simulink model "AE432_FinDel_Pioneer_WayPoint_Sim_2018a"  (R2018a)
settings: Solver=VariableStepAuto  StartTime=0  StopTime=445  FixedStep=T  RelTol=1e-3  EnableMultiTasking=on
InitFcn:
  | Waypoints
  | RollPitchTracking_Stab_ControlPioneer
values from neighbouring files (symbols this model uses):
  h = 220*ones(1,36)    [Waypoints.m]
  K1 = place(Along,Blong,P1)    [RollPitchTracking_Stab_ControlPioneer.m]
  T = 0.05    [Waypoints.m]
  x = [0 250 250 250 250 250 1250 2250 2150 2100 2050 2000 1900 1250 1250 500 500 500 500 1500 2250 2250 2250 2250 1000 1000 1000 1000 1250 1250 1250 1250 1750 1750 1750 1750]    [Waypoints.m]
  y = [0 1250 1750 2750 3500 4250 4250 4250 3750 3000 1750 1250 250 250 1500 2500 3000 3500 4000 4000 4000 3500 3000 2500 2500 3000 3500 4000 4000 3500 3000 2500 2500 3000 3500 4000]    [Waypoints.m]
undefined symbols (not defined in the file or in its folder): DiscIntNeverNeededParam, Td
libraries: simulink x19, simulink_extras x10, aerolibfltsims x2, airlib x1, aerolibanimutils x1
(part 1 of 2)
settings Model: Creator=VERBERNJ  LastModifiedBy=SHETTYA1
settings DataIOCC: SaveFormat=Array  SignalLoggingSaveFormat=ModelDataLogs  SaveOutput=off  SaveTime=off
settings OptimizationCC: BlockReduction=off  BooleanDataType=off  InitFltsAndDblsToZero=on
settings DebuggingCC: SaveWithParameterizedLinksMsg=none  UnderspecifiedInitializationDetection=Classic  MergeDetectMultiDrivingBlocksExec=none  SignalResolutionControl=TryResolveAllWithWarning  MultiTaskDSMMsg=warning  MultiTaskCondExecSysMsg=none  LibraryContextMissingDiagnostic=warning
settings HardwareCC: TargetUnknown=on
settings ModelReferenceCC: PropagateSignalLabelsOutOfModel=off
settings SFSimCC: SimUseLocalCustomCode=on
settings RTWCC: RTWUseLocalCustomCode=on
settings GRTTargetCC: TargetFcnLib=ansi_tfl_tmw.mat  TargetLangStandard=C89/C90 (ANSI)  CombineOutputUpdateFcns=off  GRTInterface=on

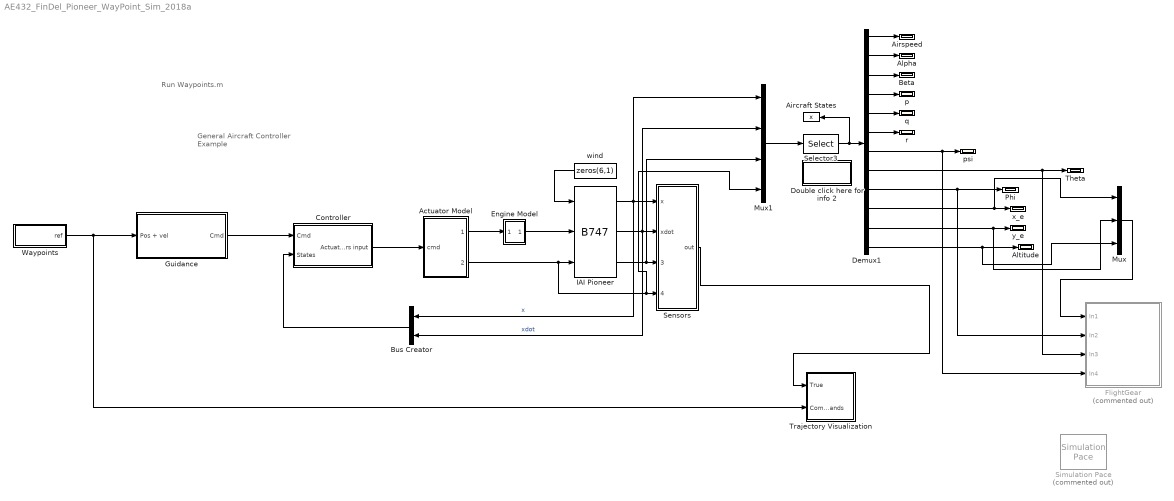
== system AE432_FinDel_Pioneer_WayPoint_Sim_2018a ==
  note: Run Waypoints.m
  note: General Aircraft
      | Controller Example
  " IAI Pioneer " : airlib/B747  GM1="[0.5486  5.1511  2.8261   47.2259  90.9483  111.4754   0  -6.6462  0   190.512]"  CD_wind="[0.060  0.430  0  0.0180  0]"  CL_wind="[0.385  4.78  8.05  0.401  0]"  Cm_body="[0.194  -2.12   -36.6   -1.76    0]"  CY_body="[0   -0.819    0     0    0.191    0]"  Cl_body="[0   -0.023   -0.450   0.265   -0.161  -0.00229]"  Cn_body="[0    0.109  -0.110  -0.200    0.0200  -0.0917]"  x0="[41.1556 0.0506 0   0 0 0   0 0.0506 0   0 0 220]"
  Actuator Model : Subsystem
  Aircraft States : ToWorkspace  VariableName=x  SampleTime=0.05
  Airspeed : Scope
  Alpha : Scope
  Altitude : Scope
  Beta : Scope
  Bus Creator : BusCreator  Inputs=2
  Controller : Subsystem
  Demux1 : Demux  Outputs=12
  Double click here for info 2 : Subsystem
      mask Display: disp('Output\nSignals')
  Engine Model : Subsystem
  FlightGear : Subsystem  Commented=on
  Guidance : Subsystem
  Mux : Mux  Inputs=3
  Mux1 : Mux  Inputs=[12 12 12 4]
  Phi : Scope
  Selector3 : Selector  InputPortWidth=40  IndexOptions=Index vector (dialog)  Indices=1:12  OutputSizes=1
  Sensors : Subsystem
  Simulation Pace : aerolibanimutils/Simulation Pace  Commented=on  SimulationPace=1  SleepMode=MATLAB Thread  OutputPaceError=off  SampleTime=Td
      settings: AttributesFormatString=%<SimulationPace> sec/sec
  Theta : Scope
  Trajectory Visualization : Subsystem
  Waypoints : Subsystem  mask(Reference Path Generation){Px=y, Py=x, Ph=h, Pt=t, T=T}
      mask prompts: Px "X Positions"; Py "Y Positions"; Ph "H Positions"; Pt "Time"; T "Sample Time"
      mask help:
      | This block generates a 3D trajectory. The output is a vector containing
      |   the position and velocity of a point that sequentially visits each X,Y,Z
      |   position at the corrisponding time. The velocity is constant between
      |   one visited point and the next.
      mask Help:
      | This block generates a 3D trajectory. The output is a vector containing
      |   the position and velocity of a point that sequentially visits each X,Y,Z
      |   position at the corrisponding time. The velocity is constant between
      |   one visited point and the next.
  p : Scope
  psi : Scope
  q : Scope
  r : Scope
  wind : Constant  Value=zeros(6,1)
  x_e : Scope
  y_e : Scope
  wires:
  " IAI Pioneer "/1 -> Mux1/1, Bus Creator/1, Sensors/1(x)  "x"
  wind/1 -> " IAI Pioneer "/1
  Actuator Model/1(Throttle) -> Engine Model/1(uprop)
  " IAI Pioneer "/2 -> Mux1/2, Bus Creator/2, Sensors/2(xdot)  "xdot"
  " IAI Pioneer "/3 -> Mux1/3, Sensors/3(others)
  Actuator Model/2(Surfaces) -> " IAI Pioneer "/3, Mux1/4, Sensors/4(controls)
  Waypoints/1(ref) -> Guidance/1(Pos + vel), Trajectory Visualization/2(Commands)
  Sensors/1(out) -> Trajectory Visualization/1(True)
  Engine Model/1(FMprop) -> " IAI Pioneer "/2
  Controller/1(Actuators input) -> Actuator Model/1(cmd)
  Guidance/1(Cmd) -> Controller/1(Cmd)
  Bus Creator/1 -> Controller/2(States)
  Demux1/12 -> Mux/3, Altitude/1
  Demux1/11 -> Mux/2, y_e/1
  Demux1/10 -> Mux/1, x_e/1
  Demux1/8 -> FlightGear/3(In3), Theta/1
  Demux1/7 -> FlightGear/4(In4), psi/1
  Demux1/6 -> r/1
  Demux1/5 -> q/1
  Demux1/4 -> p/1
  Demux1/3 -> Beta/1
  Demux1/2 -> Alpha/1
  Demux1/1 -> Airspeed/1
  Selector3/1 -> Aircraft States/1, Demux1/1
  Mux1/1 -> Selector3/1
  Demux1/9 -> Phi/1, FlightGear/2(In2)
  Mux/1 -> FlightGear/1(In1)

== system AE432_FinDel_Pioneer_WayPoint_Sim_2018a/Actuator Model ==
  cmd : Inport
  Demux : Demux  Outputs=[1 1 1 1]
  Elevator Trim : Constant  Value=0.0493
  Mux1 : Mux
  Sum5 : Sum  Inputs=++|  SaturateOnIntegerOverflow=on  InputSameDT=on  OutDataTypeStr=Inherit: Same as first input
  Thrust : Constant  Value=0.36
  flap : Constant  Value=0
  wind1 : Gain  Gain=-1  SaturateOnIntegerOverflow=on  OutDataTypeStr=Inherit: Same as input  ParamDataTypeStr=Inherit: Same as input
  wind2 : Gain  Gain=-1/3  SaturateOnIntegerOverflow=on  OutDataTypeStr=Inherit: Same as input  ParamDataTypeStr=Inherit: Same as input
  wind4 : Gain  Gain=-1/3  SaturateOnIntegerOverflow=on  OutDataTypeStr=Inherit: Same as input  ParamDataTypeStr=Inherit: Same as input
  Throttle : Outport
  Surfaces : Outport  Port=2
  wires:
  flap/1 -> Mux1/4
  cmd/1 -> Demux/1
  Mux1/1 -> Surfaces/1  "uaero"
  Demux/2 -> wind2/1
  Demux/3 -> wind4/1
  Demux/1 -> wind1/1
  Elevator Trim/1 -> Sum5/1
  Sum5/1 -> Mux1/1
  wind2/1 -> Mux1/2
  wind4/1 -> Mux1/3
  wind1/1 -> Sum5/2
  Demux/4 -> Throttle/1

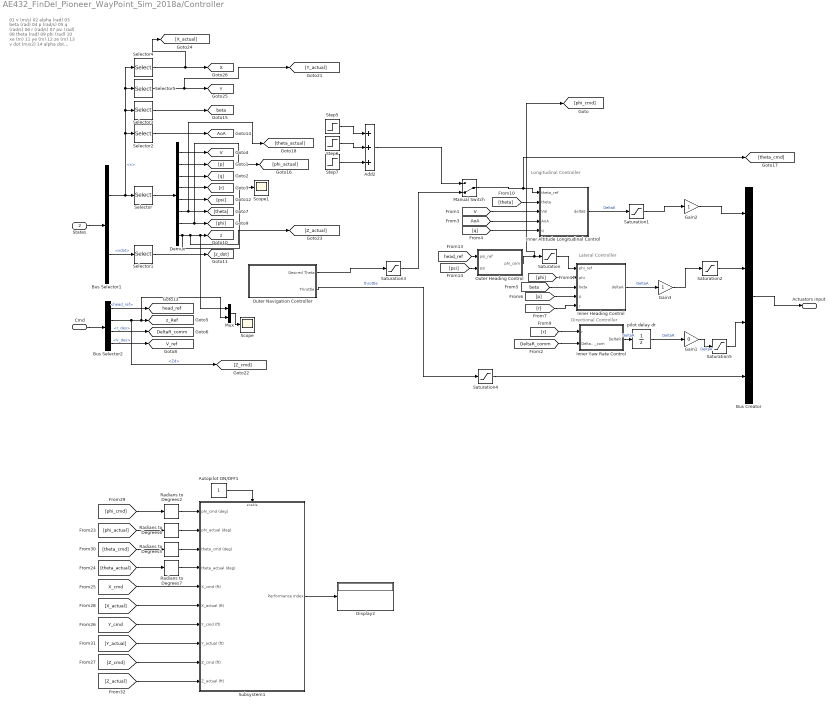
== system AE432_FinDel_Pioneer_WayPoint_Sim_2018a/Controller ==
  note: 01 v (m/s)
      | 02 alpha (rad)
      | 03 beta (rad)
      | 04 p (rad/s)
      | 05 q (rad/s)
      | 06 r  (rad/s)
      | 07 psi (rad)
      | 08 theta (rad)
      | 09 phi (rad)
      | 10 xe (m)
      | 11 ye (m)
      | 12 ze (m)
      |
      | 13 v dot (m/s2)
      | 14 alpha dot (rad/s)
      | 15 beta dot (rad/s)
      | 16 p dot (rad/s2)
      | 17 q dot (rad/s2)
      | 18 r dot (rad/s2)
      | 19 fi dot (rad/s)
      | 20 theta dot (rad/s)
      | 21 psi dot (rad/s)
      | 22 xe dot (m/s)
      | 23 ye dot (m/s)
      | 24 ze dot (m/s)
      |
      | 25 u dot (m/s2)
      | 26 v dot (m/s2)
      | 27 w dot (m/s2)
      | 28 pb/2v (rad)
      | 29 qc/v (rad)
      | 30 rb/v (rad)
      | 31 Ax (g)
      | 32 Ay (g)
      | 33 Az (g)
      | 34 ax (g)
      | 35 ay (g)
      | 36 az (g)
  note: Directional Controller
  note: Longitudinal Controller
  note: Lateral Controller
  Cmd : Inport
  States : Inport  Port=2
  Add2 : Sum  Inputs=+++
  Autopilot ON/OFF1 : Constant
  Bus Creator : BusCreator  Inputs=4
  Bus Selector1 : BusSelector  OutputSignals=x,xdot
  Bus Selector2 : BusSelector  OutputSignals=head_ref,Zd,r_des,V_des
  Demux : Demux  Outputs=8
  Display2 : Display
  Gain1 : Gain  Gain=0
  Gain2 : Gain
  Gain3 : Gain
  Inner Altitude Longitudinal Control : Subsystem  TreatAsAtomicUnit=on
  Inner Heading Control : Subsystem  TreatAsAtomicUnit=on
  Inner Yaw Rate Control : Subsystem  TreatAsAtomicUnit=on
  Manual Switch : ManualSwitch  CurrentSetting=0
  Mux : Mux  Inputs=2
  Outer Heading Control : Subsystem  TreatAsAtomicUnit=on
  Outer Navigation Controller : Subsystem
  Radians to Degrees{2,5..7} (4 alike) : simulink_extras/Transformations/Radians to Degrees
  Saturation : Saturate  UpperLimit=62*pi/180  LowerLimit=-62*pi/180
  Saturation1 : Saturate  UpperLimit=40*pi/180  LowerLimit=-40*pi/180
  Saturation2 : Saturate  UpperLimit=45*pi/180  LowerLimit=-45*pi/180
  Saturation3 : Saturate  UpperLimit=65*pi/180  LowerLimit=-65*pi/180
  Saturation4 : Saturate  UpperLimit=1  LowerLimit=0
  Saturation5 : Saturate  UpperLimit=40*pi/180  LowerLimit=-40*pi/180
  Scope : Scope
  Scope1 : Scope
  Selector : Selector  InputPortWidth=12  IndexOptions=Index vector (dialog)  Indices=[1 4 5 6 7 8 9 12]  OutputSizes=1
  Selector1 : Selector  InputPortWidth=12  IndexOptions=Index vector (dialog)  Indices=12  OutputSizes=1
  Selector2 : Selector  InputPortWidth=12  IndexOptions=Index vector (dialog)  Indices=2  OutputSizes=1
  Selector3 : Selector  InputPortWidth=12  IndexOptions=Index vector (dialog)  Indices=3  OutputSizes=1
  Selector4 : Selector  InputPortWidth=12  IndexOptions=Index vector (dialog)  Indices=10  OutputSizes=1
  Selector5 : Selector  InputPortWidth=12  IndexOptions=Index vector (dialog)  Indices=11  OutputSizes=1
  Step5 : Step  After=30*pi/180
  Step6 : Step  Time=20  Before=30*pi/180  After=-30*pi/180
  Step7 : Step  Time=40  Before=-30*pi/180  After=0
  Subsystem1 : Subsystem
  pilot delay dr : UnitDelay  SampleTime=-1
  Actuators input : Outport
  tag scope: AoA=global, DeltaR_comm=global, V=global, V_ref=global, X=global, Y=global, beta=global, head_ref=global, z=global, z_Ref=global
  wires:
  Bus Selector1/2 -> Selector1/1  "<xdot>"
  Selector/1 -> Demux/1
  Bus Selector1/1 -> Selector5/1, Selector4/1, Selector3/1, Selector2/1, Selector/1  "<x>"
  Outer Navigation Controller/2(Throttle) -> Saturation4/1  "throttle"
  pilot delay dr/1 -> Gain1/1  "DeltaR"
  Demux/1 -> [V]
  Inner Yaw Rate Control/1(DeltaR) -> pilot delay dr/1  "DeltaR"
  [DeltaR_comm] -> Inner Yaw Rate Control/2(DeltaR_com)
  [theta] -> Inner Altitude Longitudinal Control/2(theta)
  [phi] -> Inner Heading Control/2(phi)
  [psi] -> Outer Heading Control/2(psi)
  [head_ref] -> Outer Heading Control/1(psi_ref)
  Bus Selector2/4 -> [V_ref]  "<V_des>"
  Bus Selector2/3 -> [DeltaR_comm]  "<r_des>"
  Bus Selector2/2 -> [Z_cmd], Mux/2, [z_Ref]  "<Zd>"
  Bus Selector2/1 -> [head_ref]  "<head_ref>"
  Demux/5 -> [psi]
  [r] -> Inner Yaw Rate Control/1(r)
  States/1 -> Bus Selector1/1
  Selector1/1 -> [z_dot]
  Demux/8 -> Scope1/1, [Z_actual], Mux/1, [z]
  Demux/7 -> [phi_actual], [phi]
  Demux/4 -> [r]
  Demux/3 -> [q]
  Demux/2 -> [p]
  Bus Creator/1 -> Actuators input/1
  Cmd/1 -> Bus Selector2/1
  Manual Switch/1 -> [theta_cmd], Inner Altitude Longitudinal Control/1(theta_ref)
  [V] -> Inner Altitude Longitudinal Control/3(Vel)
  [AoA] -> Inner Altitude Longitudinal Control/4(AoA)
  [q] -> Inner Altitude Longitudinal Control/5(q)
  Selector2/1 -> [AoA]
  Selector3/1 -> [beta]
  Gain1/1 -> Saturation5/1  "DeltaR"
  Inner Heading Control/1(deltaA) -> Gain3/1  "DeltaA"
  Gain2/1 -> Bus Creator/1
  [beta] -> Inner Heading Control/3(beta)
  [p] -> Inner Heading Control/4(p)
  [r] -> Inner Heading Control/5(r)
  Add2/1 -> Manual Switch/1
  Step6/1 -> Add2/2
  Step5/1 -> Add2/1
  Step7/1 -> Add2/3
  Outer Heading Control/1(phi_com) -> Saturation/1, [phi_cmd]
  Saturation/1 -> Inner Heading Control/1(phi_ref)
  Saturation1/1 -> Gain2/1
  Inner Altitude Longitudinal Control/1(deltaE) -> Saturation1/1  "DeltaE"
  Saturation2/1 -> Bus Creator/2
  Gain3/1 -> Saturation2/1
  Saturation3/1 -> Manual Switch/2
  Outer Navigation Controller/1(Desired Theta) -> Saturation3/1
  Demux/6 -> [theta_actual], [theta]
  Selector5/1 -> [Y_actual], [Y]
  Selector4/1 -> [X_actual], [X]
  Mux/1 -> Scope/1
  Saturation4/1 -> Bus Creator/4
  Saturation5/1 -> Bus Creator/3
  Radians to Degrees5/1 -> Subsystem1/3(theta_cmd (deg))
  [X_actual] -> Subsystem1/6(X_actual (ft))
  Radians to Degrees7/1 -> Subsystem1/4(theta_actual (deg))
  [Y_actual] -> Subsystem1/8(Y_actual (ft))
  [Z_actual] -> Subsystem1/10(Z_actual (ft))
  [phi_cmd] -> Radians to Degrees2/1
  [phi_actual] -> Radians to Degrees6/1
  [theta_cmd] -> Radians to Degrees5/1
  [Y_cmd] -> Subsystem1/7(Y_cmd (ft))
  Radians to Degrees6/1 -> Subsystem1/2(phi_actual (deg))
  [X_cmd] -> Subsystem1/5(X_cmd (ft))
  Radians to Degrees2/1 -> Subsystem1/1(phi_cmd (deg))
  Autopilot ON/OFF1/1 -> Subsystem1/Enable
  Subsystem1/1(Performance Index) -> Display2/1
  [Z_cmd] -> Subsystem1/9(Z_cmd (ft))
  [theta_actual] -> Radians to Degrees7/1

== system AE432_FinDel_Pioneer_WayPoint_Sim_2018a/Double click here for info 2 ==
  note: 01 v (m/s)
      | 02 alpha (rad)
      | 03 beta (rad)
      | 04 p (rad/s)
      | 05 q (rad/s)
      | 06 r  (rad/s)
      | 07 psi (rad)
      | 08 theta (rad)
      | 09 phi (rad)
      | 10 xe (m)
      | 11 ye (m)
      | 12 ze (m)
      | 13 v dot (m/s2)
      | 14 alpha dot (rad/s)
      | 15 beta dot (rad/s)
      | 16 p dot (rad/s2)
      | 17 q dot (rad/s2)
      | 18 r dot (rad/s2)
      | 19 fi dot (rad/s)
      | 20 theta dot (rad/s)
      | 21 psi dot (rad/s)
      | 22 xe dot (m/s)
      | 23 ye dot (m/s)
      | 24 ze dot (m/s)
      | 25 u dot (m/s2)
      | 26 v dot (m/s2)
      | 27 w dot (m/s2)
      | 28 pb/2v (rad)
      | 29 qc/v (rad)
      | 30 rb/v (rad)
      | 31 Ax (g)
      | 32 Ay (g)
      | 33 Az (g)
      | 34 ax (g)
      | 35 ay (g)
      | 36 az (g)
      | 37 delta elevators (rad)
      | 38 delta ailerons (rad)
      | 39 delta rudder (rad)
      | 40 delta stabs (rad)

== system AE432_FinDel_Pioneer_WayPoint_Sim_2018a/Engine Model ==
  uprop : Inport
  Mux1 : Mux  Inputs=6
  const : Constant  Value=0  SampleTime=-1
  xfix : Gain  Gain=667  SaturateOnIntegerOverflow=on  OutDataTypeStr=Inherit: Same as input  ParamDataTypeStr=Inherit: Same as input
  FMprop : Outport  InitialOutput=0
  wires:
  uprop/1 -> xfix/1
  Mux1/1 -> FMprop/1
  const/1 -> Mux1/5, Mux1/4, Mux1/3, Mux1/2, Mux1/6
  xfix/1 -> Mux1/1

== system AE432_FinDel_Pioneer_WayPoint_Sim_2018a/FlightGear ==
  In1 : Inport
  In2 : Inport  Port=2
  In3 : Inport  Port=3
  In4 : Inport  Port=4
  Data Type Conversion : DataTypeConversion  OutDataTypeStr=single
  Data Type Conversion1 : DataTypeConversion  OutDataTypeStr=single
  Data Type Conversion2 : DataTypeConversion  OutDataTypeStr=single
  Lat,Lon,Elev Convertor : Subsystem
  Pack net_fdm Packet for FlightGear : aerolibfltsims/Pack net_fdm Packet for FlightGear  FlightGearVersion=v2.4  ShowPositionAttitudeInputs=on  ShowVelocityAccelerationInputs=off  ShowControlSurfacePositionInputs=off  ShowEngineFuelInputs=off  ShowLandingGearInputs=off  ShowEnvironmentInputs=off  SampleTime=-1
      settings: SourceProductName=Aerospace Blockset  SourceProductBaseCode=AE
  Send net_fdm Packet to FlightGear : aerolibfltsims/Send net_fdm Packet to FlightGear  DestinationIpAddress=127.0.0.1  DestinationPort=5502  LocalIpPort=-1  varLen=off  SampleTime=-1
      settings: SourceProductName=Aerospace Blockset  SourceProductBaseCode=AE
  wires:
  In2/1 -> Data Type Conversion2/1
  In3/1 -> Data Type Conversion1/1
  Lat,Lon,Elev Convertor/2(Lat) -> Pack net_fdm Packet for FlightGear/2
  Lat,Lon,Elev Convertor/3(Ele) -> Pack net_fdm Packet for FlightGear/3
  In1/1 -> Lat,Lon,Elev Convertor/1(Inp)
  Data Type Conversion1/1 -> Pack net_fdm Packet for FlightGear/5
  Data Type Conversion2/1 -> Pack net_fdm Packet for FlightGear/4
  Lat,Lon,Elev Convertor/1(Lon) -> Pack net_fdm Packet for FlightGear/1
  In4/1 -> Data Type Conversion/1
  Data Type Conversion/1 -> Pack net_fdm Packet for FlightGear/6
  Pack net_fdm Packet for FlightGear/1 -> Send net_fdm Packet to FlightGear/1

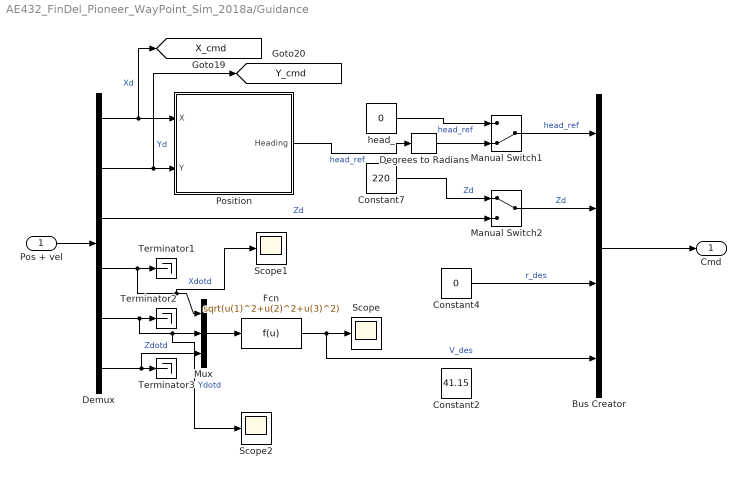
== system AE432_FinDel_Pioneer_WayPoint_Sim_2018a/Guidance ==
  Pos + vel : Inport
  Bus Creator : BusCreator  Inputs=4
  Constant2 : Constant  Value=41.15  SampleTime=-1
  Constant4 : Constant  Value=0  SampleTime=-1
  Constant7 : Constant  Value=220  SampleTime=-1
  Degrees to Radians : simulink_extras/Transformations/Degrees to Radians
  Demux : Demux  Outputs=6
  Fcn : Fcn  Expr=sqrt(u(1)^2+u(2)^2+u(3)^2)
  Manual Switch1 : ManualSwitch  CurrentSetting=0
  Manual Switch2 : ManualSwitch
  Mux : Mux  Inputs=3
  Position : Subsystem
  Scope : Scope
  Scope1 : Scope
  Scope2 : Scope
  Terminator1 : Terminator
  Terminator2 : Terminator
  Terminator3 : Terminator
  head_ : Constant  Value=0  SampleTime=-1
  Cmd : Outport
  tag scope: X_cmd=global, Y_cmd=global
  wires:
  Pos + vel/1 -> Demux/1
  Demux/3 -> Manual Switch2/2  "Zd"
  Bus Creator/1 -> Cmd/1
  Degrees to Radians/1 -> Manual Switch1/2
  head_/1 -> Manual Switch1/1  "head_ref"
  Position/1(Heading) -> Degrees to Radians/1  "head_ref"
  Demux/4 -> Scope1/1, Mux/1, Terminator1/1  "Xdotd"
  Manual Switch2/1 -> Bus Creator/2  "Zd"
  Manual Switch1/1 -> Bus Creator/1  "head_ref"
  Demux/6 -> Mux/3, Terminator3/1  "Zdotd"
  Fcn/1 -> Bus Creator/4, Scope/1  "V_des"
  Constant4/1 -> Bus Creator/3  "r_des"
  Demux/2 -> [Y_cmd], Position/2(Y)  "Yd"
  Constant7/1 -> Manual Switch2/1  "Zd"
  Demux/1 -> [X_cmd], Position/1(X)  "Xd"
  Demux/5 -> Scope2/1, Mux/2, Terminator2/1  "Ydotd"
  Mux/1 -> Fcn/1

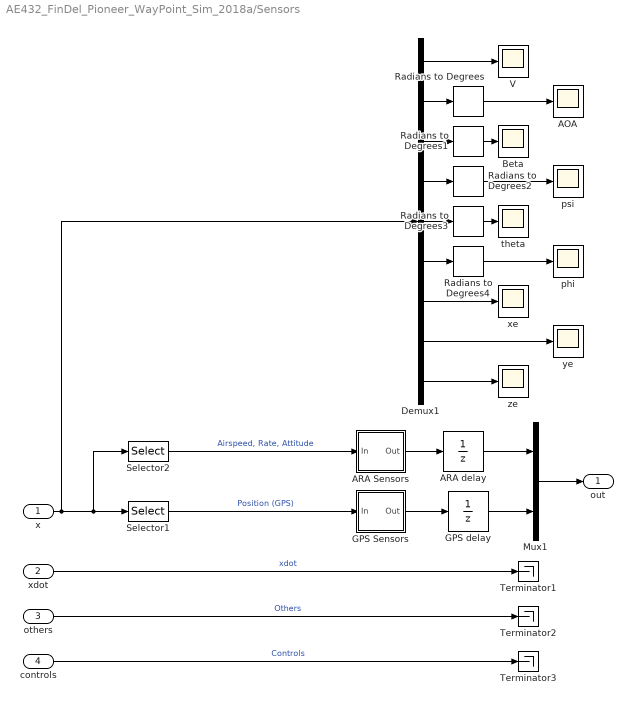
== system AE432_FinDel_Pioneer_WayPoint_Sim_2018a/Sensors ==
  x : Inport
  xdot : Inport  Port=2
  others : Inport  Port=3
  controls : Inport  Port=4
  AOA : Scope
  ARA Sensors : Subsystem
  ARA delay : UnitDelay  InitialCondition="[60 -0.0293682 0   0 0 0   0 -0.0293682 0]"  SampleTime=T
  Beta : Scope
  Demux1 : Demux  Outputs=9
  GPS Sensors : Subsystem
  GPS delay : UnitDelay  InitialCondition="[-2.5  0  60]"  SampleTime=T
  Mux1 : Mux  Inputs=[9 3]
  Radians to Degrees{,1..4} (5 alike) : simulink_extras/Transformations/Radians to Degrees
  Selector1 : Selector  InputPortWidth=12  IndexOptions=Index vector (dialog)  Indices=[10 11 12]  OutputSizes=1
  Selector2 : Selector  InputPortWidth=12  IndexOptions=Index vector (dialog)  Indices=[1:9]  OutputSizes=1
  Terminator1 : Terminator
  Terminator2 : Terminator
  Terminator3 : Terminator
  V : Scope
  phi : Scope
  psi : Scope
  theta : Scope
  xe : Scope
  ye : Scope
  ze : Scope
  out : Outport
  wires:
  controls/1 -> Terminator3/1  "Controls"
  others/1 -> Terminator2/1  "Others"
  xdot/1 -> Terminator1/1  "xdot"
  Mux1/1 -> out/1
  GPS Sensors/1(Out) -> GPS delay/1
  GPS delay/1 -> Mux1/2
  ARA delay/1 -> Mux1/1
  Selector1/1 -> GPS Sensors/1(In)  "Position (GPS)"
  ARA Sensors/1(Out) -> ARA delay/1
  Selector2/1 -> ARA Sensors/1(In)  "Airspeed, Rate, Attitude"
  x/1 -> Demux1/1, Selector2/1, Selector1/1
  Radians to Degrees1/1 -> Beta/1
  Radians to Degrees4/1 -> phi/1
  Demux1/8 -> ye/1
  Radians to Degrees2/1 -> psi/1
  Demux1/4 -> Radians to Degrees2/1
  Demux1/2 -> Radians to Degrees/1
  Demux1/9 -> ze/1
  Demux1/3 -> Radians to Degrees1/1
  Radians to Degrees/1 -> AOA/1
  Demux1/6 -> Radians to Degrees4/1
  Demux1/5 -> Radians to Degrees3/1
  Demux1/1 -> V/1
  Radians to Degrees3/1 -> theta/1
  Demux1/7 -> xe/1

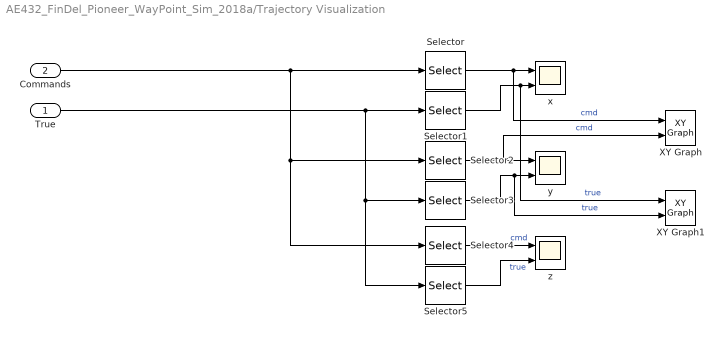
== system AE432_FinDel_Pioneer_WayPoint_Sim_2018a/Trajectory Visualization ==
  True : Inport
  Commands : Inport  Port=2
  Selector : Selector  InputPortWidth=6  IndexOptions=Index vector (dialog)  Indices=1  OutputSizes=1
  Selector1 : Selector  InputPortWidth=12  IndexOptions=Index vector (dialog)  Indices=10  OutputSizes=1
  Selector2 : Selector  InputPortWidth=6  IndexOptions=Index vector (dialog)  Indices=2  OutputSizes=1
  Selector3 : Selector  InputPortWidth=12  IndexOptions=Index vector (dialog)  Indices=11  OutputSizes=1
  Selector4 : Selector  InputPortWidth=6  IndexOptions=Index vector (dialog)  Indices=3  OutputSizes=1
  Selector5 : Selector  InputPortWidth=12  IndexOptions=Index vector (dialog)  Indices=12  OutputSizes=1
  XY Graph : simulink/Sinks/XY Graph  xmin=-100  xmax=5000  ymin=-100  ymax=3000  st=-1
  XY Graph1 : simulink/Sinks/XY Graph  xmin=-100  xmax=5000  ymin=-100  ymax=3000  st=-1
  x : Scope  NumInputPorts=2
  y : Scope  NumInputPorts=2
  z : Scope  NumInputPorts=2
  wires:
  Commands/1 -> Selector/1, Selector4/1, Selector2/1
  Selector1/1 -> XY Graph1/1, x/2  "true"
  Selector/1 -> XY Graph/1, x/1  "cmd"
  Selector2/1 -> XY Graph/2, y/1  "cmd"
  Selector3/1 -> XY Graph1/2, y/2  "true"
  Selector4/1 -> z/1  "cmd"
  Selector5/1 -> z/2  "true"
  True/1 -> Selector1/1, Selector5/1, Selector3/1

== system AE432_FinDel_Pioneer_WayPoint_Sim_2018a/Waypoints ==
  Clock : Clock
  Delay : UnitDelay  InitialCondition=[Px(1) Py(1) Ph(1)]  SampleTime=T
  Derivative : Subsystem  mask(Time Derivative){x0=[Px(1) Py(1) Ph(1)]'-[Px(2)-Px(1) Py(2)-Py(1) Ph(2)-Ph(1)]'/(Pt(2)-Pt(1))*T, T=T}
      mask prompts: x0 "Initial Condition"; T "Sampling Time"
      mask help:
      | First order approximation of the time derivative of the input signal,
      |   the original one is buggy.
  Hd(t) : Lookup  InputValues=Pt  Table=Ph  SaturateOnIntegerOverflow=on
  Horizon Time : Constant  Value=0
  Math Function : Math  Operator=mod  SaturateOnIntegerOverflow=on
  Mux : Mux  Inputs=3
  Mux2 : Mux  Inputs=[3 3]
  Sum2 : Sum  Inputs=++|  SaturateOnIntegerOverflow=on  InputSameDT=on  OutDataTypeStr=Inherit: Same as first input
  Time Limit : Constant  Value=Pt(end)
  Xd(t) : Lookup  InputValues=Pt  Table=Px  SaturateOnIntegerOverflow=on
  Yd(t) : Lookup  InputValues=Pt  Table=Py  SaturateOnIntegerOverflow=on
  ref : Outport
  wires:
  Mux2/1 -> ref/1
  Derivative/1(xdot) -> Mux2/2
  Delay/1 -> Mux2/1
  Xd(t)/1 -> Mux/1
  Yd(t)/1 -> Mux/2
  Hd(t)/1 -> Mux/3
  Sum2/1 -> Math Function/1
  Horizon Time/1 -> Sum2/1
  Clock/1 -> Sum2/2
  Math Function/1 -> Xd(t)/1, Yd(t)/1, Hd(t)/1
  Time Limit/1 -> Math Function/2
  Mux/1 -> Delay/1, Derivative/1(x)

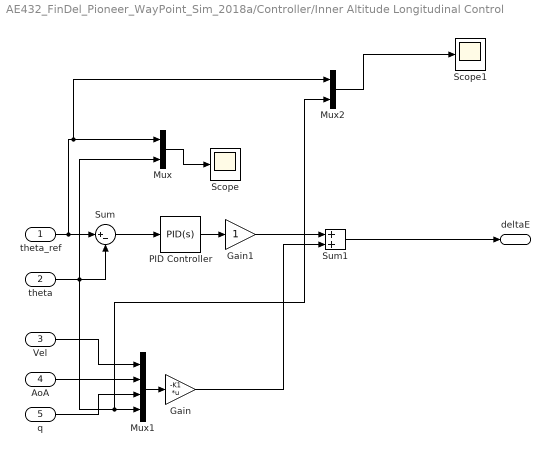
== system AE432_FinDel_Pioneer_WayPoint_Sim_2018a/Controller/Inner Altitude Longitudinal Control ==
  theta_ref : Inport
  theta : Inport  Port=2
  Vel : Inport  Port=3
  AoA : Inport  Port=4
  q : Inport  Port=5
  Gain : Gain  Gain=-K1  Multiplication=Matrix(K*u)
  Gain1 : Gain
  Mux : Mux  Inputs=2
  Mux1 : Mux
  Mux2 : Mux  Inputs=2
  PID Controller : simulink/Continuous/PID Controller  Controller=PID  TimeDomain=Continuous-time  SampleTime=-1  IntegratorMethod=Forward Euler  FilterMethod=Forward Euler  Form=Parallel  UseFilter=on  ControllerParametersSource=internal  P=3.5  I=0.7  D=0.001  N=50  InitialConditionSource=internal  InitialConditionForIntegrator=0  InitialConditionForFilter=0  ExternalReset=none  LimitOutput=off  UpperSaturationLimit=inf  LowerSaturationLimit=-inf  LinearizeAsGain=on  AntiWindupMode=none  Kb=1  TrackingMode=off  Kt=1  PParamMin=[]  PParamMax=[]  IParamMin=[]  IParamMax=[]  DParamMin=[]  DParamMax=[]  NParamMin=[]  NParamMax=[]  KbParamMin=[]  KbParamMax=[]  KtParamMin=[]  KtParamMax=[]  POutMin=[]  POutMax=[]  IOutMin=[]  IOutMax=[]  DOutMin=[]  DOutMax=[]  NOutMin=[]  NOutMax=[]  KbOutMin=[]  KbOutMax=[]  KtOutMin=[]  KtOutMax=[]  IntegratorOutMin=[]  IntegratorOutMax=[]  FilterOutMin=[]  FilterOutMax=[]  SumOutMin=[]  SumOutMax=[]  SumI1OutMin=[]  SumI1OutMax=[]  SumI2OutMin=[]  SumI2OutMax=[]  SumI3OutMin=[]  SumI3OutMax=[]  SumDOutMin=[]  SumDOutMax=[]  SaturationOutMin=[]  SaturationOutMax=[]  IntegratorContinuousStateAttributes=''  IntegratorStateMustResolveToSignalObject=off  IntegratorRTWStateStorageClass=Auto  FilterContinuousStateAttributes=''  FilterStateMustResolveToSignalObject=off  FilterRTWStateStorageClass=Auto  DifferentiatorICPrevScaledInput=0  DifferentiatorOutMin=[]  DifferentiatorOutMax=[]  FilterDiffOutCoefMin=[]  FilterDiffOutCoefMax=[]  SumDenOutMin=[]  SumDenOutMax=[]  SumNumOutMin=[]  SumNumOutMax=[]  ReciprocalOutMin=[]  ReciprocalOutMax=[]  DivideOutMin=[]  DivideOutMax=[]  TunerSelectOption=Transfer Function Based (PID Tuner App)
  Scope : Scope
  Scope1 : Scope
  Sum : Sum  Inputs=|+-
  Sum1 : Sum
  deltaE : Outport
  wires:
  theta/1 -> Mux2/2, Mux1/4, Mux/2, Sum/2
  Sum/1 -> PID Controller/1
  Mux/1 -> Scope/1
  theta_ref/1 -> Mux2/1, Mux/1, Sum/1
  Vel/1 -> Mux1/1
  AoA/1 -> Mux1/2
  q/1 -> Mux1/3
  Mux1/1 -> Gain/1
  PID Controller/1 -> Gain1/1
  Sum1/1 -> deltaE/1
  Gain1/1 -> Sum1/1
  Gain/1 -> Sum1/2
  Mux2/1 -> Scope1/1

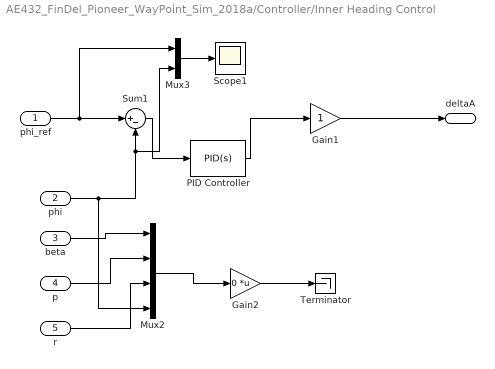
== system AE432_FinDel_Pioneer_WayPoint_Sim_2018a/Controller/Inner Heading Control ==
  phi_ref : Inport
  phi : Inport  Port=2
  beta : Inport  Port=3
  p : Inport  Port=4
  r : Inport  Port=5
  Gain1 : Gain
  Gain2 : Gain  Gain=0  Multiplication=Matrix(K*u)
  Mux2 : Mux
  Mux3 : Mux  Inputs=2
  PID Controller : simulink/Continuous/PID Controller  Controller=PID  TimeDomain=Continuous-time  SampleTime=-1  IntegratorMethod=Forward Euler  FilterMethod=Forward Euler  Form=Parallel  UseFilter=on  ControllerParametersSource=internal  P=2  I=0.355  D=0.025  N=20  InitialConditionSource=internal  InitialConditionForIntegrator=0  InitialConditionForFilter=0  ExternalReset=none  LimitOutput=off  UpperSaturationLimit=inf  LowerSaturationLimit=-inf  LinearizeAsGain=on  AntiWindupMode=none  Kb=1  TrackingMode=off  Kt=1  PParamMin=[]  PParamMax=[]  IParamMin=[]  IParamMax=[]  DParamMin=[]  DParamMax=[]  NParamMin=[]  NParamMax=[]  KbParamMin=[]  KbParamMax=[]  KtParamMin=[]  KtParamMax=[]  POutMin=[]  POutMax=[]  IOutMin=[]  IOutMax=[]  DOutMin=[]  DOutMax=[]  NOutMin=[]  NOutMax=[]  KbOutMin=[]  KbOutMax=[]  KtOutMin=[]  KtOutMax=[]  IntegratorOutMin=[]  IntegratorOutMax=[]  FilterOutMin=[]  FilterOutMax=[]  SumOutMin=[]  SumOutMax=[]  SumI1OutMin=[]  SumI1OutMax=[]  SumI2OutMin=[]  SumI2OutMax=[]  SumI3OutMin=[]  SumI3OutMax=[]  SumDOutMin=[]  SumDOutMax=[]  SaturationOutMin=[]  SaturationOutMax=[]  IntegratorContinuousStateAttributes=''  IntegratorStateMustResolveToSignalObject=off  IntegratorRTWStateStorageClass=Auto  FilterContinuousStateAttributes=''  FilterStateMustResolveToSignalObject=off  FilterRTWStateStorageClass=Auto  DifferentiatorICPrevScaledInput=0  DifferentiatorOutMin=[]  DifferentiatorOutMax=[]  FilterDiffOutCoefMin=[]  FilterDiffOutCoefMax=[]  SumDenOutMin=[]  SumDenOutMax=[]  SumNumOutMin=[]  SumNumOutMax=[]  ReciprocalOutMin=[]  ReciprocalOutMax=[]  DivideOutMin=[]  DivideOutMax=[]  TunerSelectOption=Transfer Function Based (PID Tuner App)
  Scope1 : Scope
  Sum1 : Sum  Inputs=|+-
  Terminator : Terminator
  deltaA : Outport
  wires:
  phi/1 -> Mux2/4, Mux3/2, Sum1/2
  PID Controller/1 -> Gain1/1
  Sum1/1 -> PID Controller/1
  phi_ref/1 -> Mux3/1, Sum1/1
  Mux3/1 -> Scope1/1
  beta/1 -> Mux2/1
  p/1 -> Mux2/2
  r/1 -> Mux2/3
  Mux2/1 -> Gain2/1
  Gain1/1 -> deltaA/1
  Gain2/1 -> Terminator/1

== system AE432_FinDel_Pioneer_WayPoint_Sim_2018a/Controller/Inner Yaw Rate Control ==
  r : Inport
  DeltaR_com : Inport  Port=2
  Gain : Gain
  Mux : Mux  Inputs=2
  PID Controller : simulink/Continuous/PID Controller  Controller=PID  TimeDomain=Continuous-time  SampleTime=-1  IntegratorMethod=Forward Euler  FilterMethod=Forward Euler  Form=Parallel  UseFilter=on  ControllerParametersSource=internal  P=0.002  I=0  D=0  N=50  InitialConditionSource=internal  InitialConditionForIntegrator=0  InitialConditionForFilter=0  ExternalReset=none  LimitOutput=off  UpperSaturationLimit=inf  LowerSaturationLimit=-inf  LinearizeAsGain=on  AntiWindupMode=none  Kb=1  TrackingMode=off  Kt=1  PParamMin=[]  PParamMax=[]  IParamMin=[]  IParamMax=[]  DParamMin=[]  DParamMax=[]  NParamMin=[]  NParamMax=[]  KbParamMin=[]  KbParamMax=[]  KtParamMin=[]  KtParamMax=[]  POutMin=[]  POutMax=[]  IOutMin=[]  IOutMax=[]  DOutMin=[]  DOutMax=[]  NOutMin=[]  NOutMax=[]  KbOutMin=[]  KbOutMax=[]  KtOutMin=[]  KtOutMax=[]  IntegratorOutMin=[]  IntegratorOutMax=[]  FilterOutMin=[]  FilterOutMax=[]  SumOutMin=[]  SumOutMax=[]  SumI1OutMin=[]  SumI1OutMax=[]  SumI2OutMin=[]  SumI2OutMax=[]  SumI3OutMin=[]  SumI3OutMax=[]  SumDOutMin=[]  SumDOutMax=[]  SaturationOutMin=[]  SaturationOutMax=[]  IntegratorContinuousStateAttributes=''  IntegratorStateMustResolveToSignalObject=off  IntegratorRTWStateStorageClass=Auto  FilterContinuousStateAttributes=''  FilterStateMustResolveToSignalObject=off  FilterRTWStateStorageClass=Auto  DifferentiatorICPrevScaledInput=0  DifferentiatorOutMin=[]  DifferentiatorOutMax=[]  FilterDiffOutCoefMin=[]  FilterDiffOutCoefMax=[]  SumDenOutMin=[]  SumDenOutMax=[]  SumNumOutMin=[]  SumNumOutMax=[]  ReciprocalOutMin=[]  ReciprocalOutMax=[]  DivideOutMin=[]  DivideOutMax=[]  TunerSelectOption=Transfer Function Based (PID Tuner App)
  Scope{,1..3} (4 alike) : Scope
  Sum : Sum  Inputs=|+-
  DeltaR : Outport
  wires:
  Sum/1 -> PID Controller/1
  PID Controller/1 -> Sum/2, Gain/1, Scope1/1
  Mux/1 -> Scope/1
  r/1 -> Scope2/1, Mux/1, Sum/1
  DeltaR_com/1 -> Scope3/1, Mux/2
  Gain/1 -> DeltaR/1

== system AE432_FinDel_Pioneer_WayPoint_Sim_2018a/Controller/Outer Heading Control ==
  psi_ref : Inport
  psi : Inport  Port=2
  Mux : Mux  Inputs=2
  PID Controller : simulink/Continuous/PID Controller  Controller=PID  TimeDomain=Continuous-time  SampleTime=-1  IntegratorMethod=Forward Euler  FilterMethod=Forward Euler  Form=Parallel  UseFilter=on  ControllerParametersSource=internal  P=1.574  I=.141  D=.004  N=20  InitialConditionSource=internal  InitialConditionForIntegrator=0  InitialConditionForFilter=0  ExternalReset=none  LimitOutput=off  UpperSaturationLimit=inf  LowerSaturationLimit=-inf  LinearizeAsGain=on  AntiWindupMode=none  Kb=1  TrackingMode=off  Kt=1  PParamMin=[]  PParamMax=[]  IParamMin=[]  IParamMax=[]  DParamMin=[]  DParamMax=[]  NParamMin=[]  NParamMax=[]  KbParamMin=[]  KbParamMax=[]  KtParamMin=[]  KtParamMax=[]  POutMin=[]  POutMax=[]  IOutMin=[]  IOutMax=[]  DOutMin=[]  DOutMax=[]  NOutMin=[]  NOutMax=[]  KbOutMin=[]  KbOutMax=[]  KtOutMin=[]  KtOutMax=[]  IntegratorOutMin=[]  IntegratorOutMax=[]  FilterOutMin=[]  FilterOutMax=[]  SumOutMin=[]  SumOutMax=[]  SumI1OutMin=[]  SumI1OutMax=[]  SumI2OutMin=[]  SumI2OutMax=[]  SumI3OutMin=[]  SumI3OutMax=[]  SumDOutMin=[]  SumDOutMax=[]  SaturationOutMin=[]  SaturationOutMax=[]  IntegratorContinuousStateAttributes=''  IntegratorStateMustResolveToSignalObject=off  IntegratorRTWStateStorageClass=Auto  FilterContinuousStateAttributes=''  FilterStateMustResolveToSignalObject=off  FilterRTWStateStorageClass=Auto  DifferentiatorICPrevScaledInput=0  DifferentiatorOutMin=[]  DifferentiatorOutMax=[]  FilterDiffOutCoefMin=[]  FilterDiffOutCoefMax=[]  SumDenOutMin=[]  SumDenOutMax=[]  SumNumOutMin=[]  SumNumOutMax=[]  ReciprocalOutMin=[]  ReciprocalOutMax=[]  DivideOutMin=[]  DivideOutMax=[]  TunerSelectOption=Transfer Function Based (PID Tuner App)
  Scope : Scope
  Sum : Sum  Inputs=|+-
  phi_com : Outport
  wires:
  PID Controller/1 -> phi_com/1
  Sum/1 -> PID Controller/1
  psi/1 -> Mux/2, Sum/2
  psi_ref/1 -> Mux/1, Sum/1
  Mux/1 -> Scope/1

== system AE432_FinDel_Pioneer_WayPoint_Sim_2018a/Controller/Outer Navigation Controller ==
  Outer and Inner Longitudinal Control : Subsystem  TreatAsAtomicUnit=on
  Desired Theta : Outport
  Throttle : Outport  Port=2
  wires:
  [z] -> Outer and Inner Longitudinal Control/2(Alt)
  [z_Ref] -> Outer and Inner Longitudinal Control/1(Alt_ref)
  [V_ref] -> Outer and Inner Longitudinal Control/3(V_ref)
  [V] -> Outer and Inner Longitudinal Control/4(V)
  Outer and Inner Longitudinal Control/2(Throttle) -> Throttle/1  "Throttle"
  Outer and Inner Longitudinal Control/1(theta_com) -> Desired Theta/1

== system AE432_FinDel_Pioneer_WayPoint_Sim_2018a/Controller/Subsystem1 ==
  phi_cmd (deg) : Inport
  phi_actual (deg) : Inport  Port=2
  theta_cmd (deg) : Inport  Port=3
  theta_actual (deg) : Inport  Port=4
  X_cmd (ft) : Inport  Port=5
  X_actual (ft) : Inport  Port=6
  Y_cmd (ft) : Inport  Port=7
  Y_actual (ft) : Inport  Port=8
  Z_cmd (ft) : Inport  Port=9
  Z_actual (ft) : Inport  Port=10
  Enable : EnablePort
  Performance Metrics : Subsystem
  Performance Index : Outport
  wires:
  X_cmd (ft)/1 -> Performance Metrics/5(X_cmd (ft))
  Z_cmd (ft)/1 -> Performance Metrics/9(Z_cmd (ft))
  Z_actual (ft)/1 -> Performance Metrics/10(Z_actual (ft))
  X_actual (ft)/1 -> Performance Metrics/6(X_actual (ft))
  phi_cmd (deg)/1 -> Performance Metrics/1(phi_cmd (deg))
  Y_actual (ft)/1 -> Performance Metrics/8(Y_actual (ft))
  phi_actual (deg)/1 -> Performance Metrics/2(phi_actual (deg))
  theta_cmd (deg)/1 -> Performance Metrics/3(theta_cmd (deg))
  theta_actual (deg)/1 -> Performance Metrics/4(theta_actual (deg))
  Y_cmd (ft)/1 -> Performance Metrics/7(Y_cmd (ft))
  Performance Metrics/1(Performance Index) -> Performance Index/1

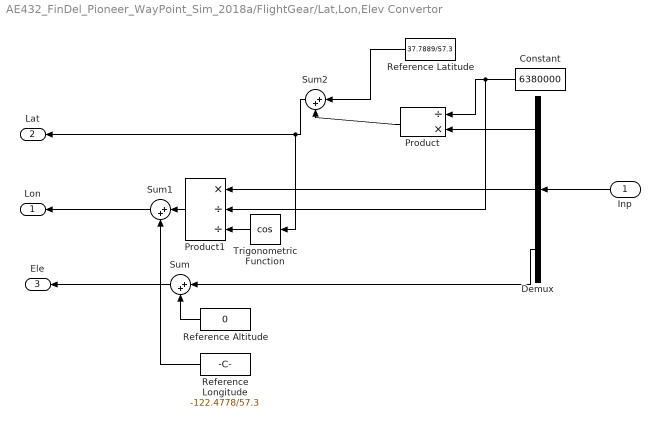
== system AE432_FinDel_Pioneer_WayPoint_Sim_2018a/FlightGear/Lat,Lon,Elev Convertor ==
  Inp : Inport
  Constant : Constant  Value=6380000
  Demux : Demux  Outputs=3
  Product : Product  Inputs=/*  SampleTime=Td  SaturateOnIntegerOverflow=on  OutDataTypeStr=Inherit: Same as first input
  Product1 : Product  Inputs=*//  SampleTime=Td  SaturateOnIntegerOverflow=on  OutDataTypeStr=Inherit: Same as first input
  Reference Altitude : Constant  Value=0
  Reference Latitude : Constant  Value=37.7889/57.3
  Reference Longitude : Constant  Value=-122.4778/57.3
  Sum : Sum  Inputs=|++  SampleTime=Td  SaturateOnIntegerOverflow=on
  Sum1 : Sum  Inputs=|++  SampleTime=Td  SaturateOnIntegerOverflow=on
  Sum2 : Sum  Inputs=|++  SampleTime=Td  SaturateOnIntegerOverflow=on
  Trigonometric Function : Trigonometry  Operator=cos  SampleTime=Td
  Lon : Outport
  Lat : Outport  Port=2
  Ele : Outport  Port=3
  wires:
  Reference Latitude/1 -> Sum2/1
  Sum1/1 -> Lon/1
  Reference Longitude/1 -> Sum1/2
  Product1/1 -> Sum1/1
  Trigonometric Function/1 -> Product1/3
  Demux/2 -> Product1/1
  Demux/3 -> Sum/1
  Sum2/1 -> Lat/1, Trigonometric Function/1
  Product/1 -> Sum2/2
  Demux/1 -> Product/2
  Constant/1 -> Product1/2, Product/1
  Reference Altitude/1 -> Sum/2
  Sum/1 -> Ele/1
  Inp/1 -> Demux/1

== system AE432_FinDel_Pioneer_WayPoint_Sim_2018a/Guidance/Position ==
  note: From XY to Heading
  X : Inport
  Y : Inport  Port=2
  Mux1 : Mux
  Mux2 : Mux  Inputs=2
  S-Function1 : S-Function  FunctionName=XYtoHeadingCorr  SFunctionDeploymentMode=off  EnableBusSupport=off  mask(S-function: XYtoHeading){}
      mask help:
      | This is a Matlab S-function that converts
      | cartesian coordinates XY to heading angle.
      | North : 0deg
      | South : 180deg
      | East: 90deg
      | West: 270deg
      |
      | X-North
      | Y-East
      mask Display:
      | plot([0 1 2 3 4 5 6 6 5 4 3 2 1 0 0],[0 0 0 0 0 0 0 6 6 6 6 6 6 6 0]);
      | disp(' Heading angle Correction');
  S-Function11 : S-Function  FunctionName=XYtoHeading  SFunctionDeploymentMode=off  EnableBusSupport=off  mask(S-function: XYtoHeading){}
      mask help:
      | This is a Matlab S-function that converts
      | cartesian coordinates XY to heading angle.
      | North : 0deg
      | South : 180deg
      | East: 90deg
      | West: 270deg
      |
      | X-North
      | Y-East
      mask Display:
      | plot([0 1 2 3 4 5 6 6 5 4 3 2 1 0 0],[0 0 0 0 0 0 0 6 6 6 6 6 6 6 0]);
      | disp('  XY to Heading angle');
  Unit Delay1 : UnitDelay  SampleTime=-1
  Unit Delay2 : UnitDelay  SampleTime=-1
  Unit Delay3 : UnitDelay  SampleTime=-1
  Heading : Outport
  wires:
  Unit Delay3/1 -> Mux2/1
  S-Function11/1 -> Mux2/2
  Mux2/1 -> S-Function1/1
  S-Function1/1 -> Unit Delay3/1, Heading/1
  Mux1/1 -> S-Function11/1
  Y/1 -> Mux1/4, Unit Delay2/1
  X/1 -> Mux1/2, Unit Delay1/1
  Unit Delay1/1 -> Mux1/1
  Unit Delay2/1 -> Mux1/3

== system AE432_FinDel_Pioneer_WayPoint_Sim_2018a/Sensors/ARA Sensors ==
  note: Insert ARA (Airspeed, Rate, Attitude) Sensors Model Here
      | ( Transfer Functions + Limiters + Noise)
  In : Inport
  Demux : Demux  Outputs=9
  Mux1 : Mux  Inputs=9
  Out : Outport
  wires:
  Demux/7 -> Mux1/7
  In/1 -> Demux/1
  Mux1/1 -> Out/1
  Demux/1 -> Mux1/1
  Demux/2 -> Mux1/2
  Demux/3 -> Mux1/3
  Demux/4 -> Mux1/4
  Demux/5 -> Mux1/5
  Demux/6 -> Mux1/6
  Demux/8 -> Mux1/8
  Demux/9 -> Mux1/9

== system AE432_FinDel_Pioneer_WayPoint_Sim_2018a/Sensors/GPS Sensors ==
  note: Add GPS Noine Model Here
  In : Inport
  Out : Outport
  wires:
  In/1 -> Out/1

== system AE432_FinDel_Pioneer_WayPoint_Sim_2018a/Waypoints/Derivative ==
  x : Inport
  Product2 : Product  Inputs=/*  SaturateOnIntegerOverflow=on  RndMeth=Zero  InputSameDT=on  OutDataTypeStr=Inherit: Same as first input
  Sum4 : Sum  Inputs=|+-  SaturateOnIntegerOverflow=on  InputSameDT=on  OutDataTypeStr=Inherit: Same as first input
  Unit Delay1 : UnitDelay  InitialCondition=x0  SampleTime=T
  Zero-Order Hold1 : ZeroOrderHold  SampleTime=T
  m : Constant  Value=T
  xdot : Outport
  wires:
  x/1 -> Zero-Order Hold1/1
  Product2/1 -> xdot/1
  m/1 -> Product2/1
  Zero-Order Hold1/1 -> Unit Delay1/1, Sum4/1
  Unit Delay1/1 -> Sum4/2
  Sum4/1 -> Product2/2

== system AE432_FinDel_Pioneer_WayPoint_Sim_2018a/Controller/Outer Navigation Controller/Outer and Inner Longitudinal Control ==
  Alt_ref : Inport
  Alt : Inport  Port=2
  V_ref : Inport  Port=3
  V : Inport  Port=4
  Inner Longitudinal Airspeed Control : Subsystem  TreatAsAtomicUnit=on
  Outer Longitudinal Altitude Control : Subsystem  TreatAsAtomicUnit=on
  theta_com : Outport
  Throttle : Outport  Port=2
  wires:
  Inner Longitudinal Airspeed Control/1(Throttle) -> Throttle/1
  Outer Longitudinal Altitude Control/1(theta_com) -> theta_com/1
  Alt/1 -> Outer Longitudinal Altitude Control/2(Alt)
  Alt_ref/1 -> Outer Longitudinal Altitude Control/1(Alt_ref)
  V/1 -> Inner Longitudinal Airspeed Control/2(V)
  V_ref/1 -> Inner Longitudinal Airspeed Control/1(V_ref)

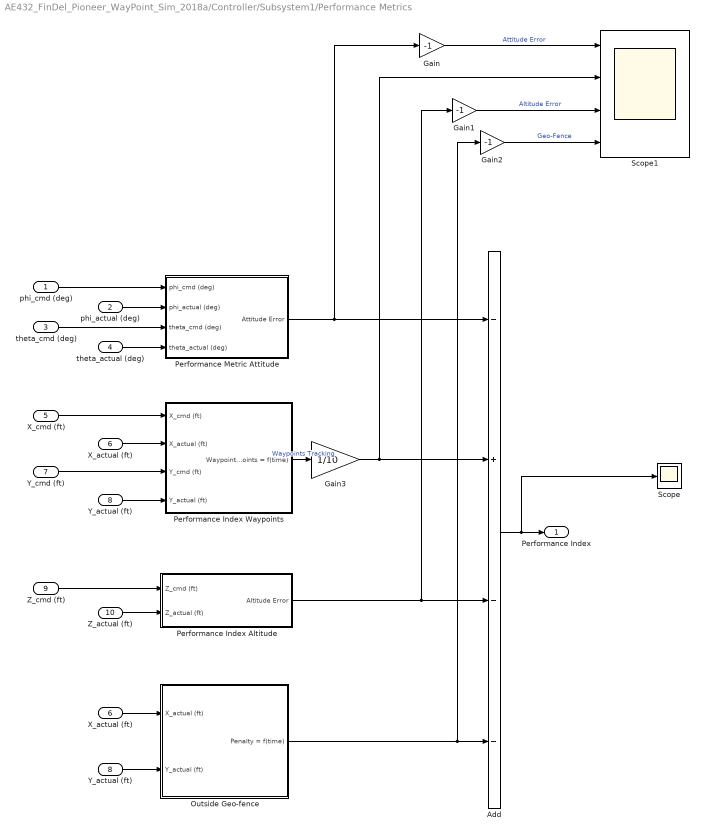
== system AE432_FinDel_Pioneer_WayPoint_Sim_2018a/Controller/Subsystem1/Performance Metrics ==
  phi_cmd (deg) : Inport
  phi_actual (deg) : Inport  Port=2
  theta_cmd (deg) : Inport  Port=3
  theta_actual (deg) : Inport  Port=4
  X_cmd (ft) : Inport  Port=5
  X_actual (ft) : Inport  Port=6
  Y_cmd (ft) : Inport  Port=7
  Y_actual (ft) : Inport  Port=8
  Z_cmd (ft) : Inport  Port=9
  Z_actual (ft) : Inport  Port=10
  Add : Sum  Inputs=-+--
  Gain : Gain  Gain=-1
  Gain1 : Gain  Gain=-1
  Gain2 : Gain  Gain=-1
  Gain3 : Gain  Gain=1/10
  Outside Geo-fence : Subsystem
  Performance Index Altitude : Subsystem
  Performance Index Waypoints : Subsystem
  Performance Metric Attitude : Subsystem
  Scope : Scope
  Scope1 : Scope  NumInputPorts=4
  "X_actual (ft) " : InportShadow  Port=6
  "Y_actual (ft) " : InportShadow  Port=8
  Performance Index : Outport
  wires:
  phi_cmd (deg)/1 -> Performance Metric Attitude/1(phi_cmd (deg))
  phi_actual (deg)/1 -> Performance Metric Attitude/2(phi_actual (deg))
  theta_cmd (deg)/1 -> Performance Metric Attitude/3(theta_cmd (deg))
  theta_actual (deg)/1 -> Performance Metric Attitude/4(theta_actual (deg))
  Z_cmd (ft)/1 -> Performance Index Altitude/1(Z_cmd (ft))
  Z_actual (ft)/1 -> Performance Index Altitude/2(Z_actual (ft))
  X_cmd (ft)/1 -> Performance Index Waypoints/1(X_cmd (ft))
  X_actual (ft)/1 -> Performance Index Waypoints/2(X_actual (ft))
  Y_actual (ft)/1 -> Performance Index Waypoints/4(Y_actual (ft))
  Y_cmd (ft)/1 -> Performance Index Waypoints/3(Y_cmd (ft))
  Performance Metric Attitude/1(Attitude Error) -> Add/1, Gain/1
  Performance Index Waypoints/1(Waypoint Points = f(time)) -> Gain3/1  "Waypoints Tracking"
  Performance Index Altitude/1(Altitude Error) -> Gain1/1, Add/3
  Add/1 -> Scope/1, Performance Index/1
  Outside Geo-fence/1(Penalty = f(time)) -> Gain2/1, Add/4
  "X_actual (ft) "/1 -> Outside Geo-fence/1(X_actual (ft))
  "Y_actual (ft) "/1 -> Outside Geo-fence/2(Y_actual (ft))
  Gain/1 -> Scope1/1  "Attitude Error"
  Gain1/1 -> Scope1/3  "Altitude Error"
  Gain2/1 -> Scope1/4  "Geo-Fence"
  Gain3/1 -> Scope1/2, Add/2

== system AE432_FinDel_Pioneer_WayPoint_Sim_2018a/Controller/Outer Navigation Controller/Outer and Inner Longitudinal Control/Inner Longitudinal Airspeed Control ==
  V_ref : Inport
  V : Inport  Port=2
  Mux : Mux  Inputs=2
  PID Controller : simulink/Continuous/PID Controller  Controller=PID  TimeDomain=Continuous-time  SampleTime=-1  IntegratorMethod=Forward Euler  FilterMethod=Forward Euler  Form=Parallel  UseFilter=on  ControllerParametersSource=internal  P=3  I=0.4  D=0.001  N=20  InitialConditionSource=internal  InitialConditionForIntegrator=0  InitialConditionForFilter=0  ExternalReset=none  LimitOutput=off  UpperSaturationLimit=inf  LowerSaturationLimit=-inf  LinearizeAsGain=on  AntiWindupMode=none  Kb=1  TrackingMode=off  Kt=1  PParamMin=[]  PParamMax=[]  IParamMin=[]  IParamMax=[]  DParamMin=[]  DParamMax=[]  NParamMin=[]  NParamMax=[]  KbParamMin=[]  KbParamMax=[]  KtParamMin=[]  KtParamMax=[]  POutMin=[]  POutMax=[]  IOutMin=[]  IOutMax=[]  DOutMin=[]  DOutMax=[]  NOutMin=[]  NOutMax=[]  KbOutMin=[]  KbOutMax=[]  KtOutMin=[]  KtOutMax=[]  IntegratorOutMin=[]  IntegratorOutMax=[]  FilterOutMin=[]  FilterOutMax=[]  SumOutMin=[]  SumOutMax=[]  SumI1OutMin=[]  SumI1OutMax=[]  SumI2OutMin=[]  SumI2OutMax=[]  SumI3OutMin=[]  SumI3OutMax=[]  SumDOutMin=[]  SumDOutMax=[]  SaturationOutMin=[]  SaturationOutMax=[]  IntegratorContinuousStateAttributes=''  IntegratorStateMustResolveToSignalObject=off  IntegratorRTWStateStorageClass=Auto  FilterContinuousStateAttributes=''  FilterStateMustResolveToSignalObject=off  FilterRTWStateStorageClass=Auto  DifferentiatorICPrevScaledInput=0  DifferentiatorOutMin=[]  DifferentiatorOutMax=[]  FilterDiffOutCoefMin=[]  FilterDiffOutCoefMax=[]  SumDenOutMin=[]  SumDenOutMax=[]  SumNumOutMin=[]  SumNumOutMax=[]  ReciprocalOutMin=[]  ReciprocalOutMax=[]  DivideOutMin=[]  DivideOutMax=[]  TunerSelectOption=Transfer Function Based (PID Tuner App)
  Scope : Scope
  Scope1 : Scope
  Scope2 : Scope
  Sum : Sum  Inputs=|+-
  Throttle : Outport
  wires:
  PID Controller/1 -> Scope1/1, Throttle/1
  Mux/1 -> Scope/1
  V/1 -> Mux/2, Sum/2
  V_ref/1 -> Scope2/1, Mux/1, Sum/1
  Sum/1 -> PID Controller/1

== system AE432_FinDel_Pioneer_WayPoint_Sim_2018a/Controller/Outer Navigation Controller/Outer and Inner Longitudinal Control/Outer Longitudinal Altitude Control ==
  Alt_ref : Inport
  Alt : Inport  Port=2
  Mux : Mux  Inputs=2
  PID Controller : simulink/Continuous/PID Controller  Controller=PID  TimeDomain=Continuous-time  SampleTime=-1  IntegratorMethod=Forward Euler  FilterMethod=Forward Euler  Form=Parallel  UseFilter=on  ControllerParametersSource=internal  P=0.45  I=0.2  D=0.05  N=50  InitialConditionSource=internal  InitialConditionForIntegrator=0  InitialConditionForFilter=0  ExternalReset=none  LimitOutput=off  UpperSaturationLimit=inf  LowerSaturationLimit=-inf  LinearizeAsGain=on  AntiWindupMode=none  Kb=1  TrackingMode=off  Kt=1  PParamMin=[]  PParamMax=[]  IParamMin=[]  IParamMax=[]  DParamMin=[]  DParamMax=[]  NParamMin=[]  NParamMax=[]  KbParamMin=[]  KbParamMax=[]  KtParamMin=[]  KtParamMax=[]  POutMin=[]  POutMax=[]  IOutMin=[]  IOutMax=[]  DOutMin=[]  DOutMax=[]  NOutMin=[]  NOutMax=[]  KbOutMin=[]  KbOutMax=[]  KtOutMin=[]  KtOutMax=[]  IntegratorOutMin=[]  IntegratorOutMax=[]  FilterOutMin=[]  FilterOutMax=[]  SumOutMin=[]  SumOutMax=[]  SumI1OutMin=[]  SumI1OutMax=[]  SumI2OutMin=[]  SumI2OutMax=[]  SumI3OutMin=[]  SumI3OutMax=[]  SumDOutMin=[]  SumDOutMax=[]  SaturationOutMin=[]  SaturationOutMax=[]  IntegratorContinuousStateAttributes=''  IntegratorStateMustResolveToSignalObject=off  IntegratorRTWStateStorageClass=Auto  FilterContinuousStateAttributes=''  FilterStateMustResolveToSignalObject=off  FilterRTWStateStorageClass=Auto  DifferentiatorICPrevScaledInput=0  DifferentiatorOutMin=[]  DifferentiatorOutMax=[]  FilterDiffOutCoefMin=[]  FilterDiffOutCoefMax=[]  SumDenOutMin=[]  SumDenOutMax=[]  SumNumOutMin=[]  SumNumOutMax=[]  ReciprocalOutMin=[]  ReciprocalOutMax=[]  DivideOutMin=[]  DivideOutMax=[]  TunerSelectOption=Transfer Function Based (PID Tuner App)
  Scope : Scope
  Sum : Sum  Inputs=|+-
  theta_com : Outport
  wires:
  Mux/1 -> Scope/1
  PID Controller/1 -> theta_com/1
  Sum/1 -> PID Controller/1
  Alt/1 -> Mux/2, Sum/2
  Alt_ref/1 -> Mux/1, Sum/1

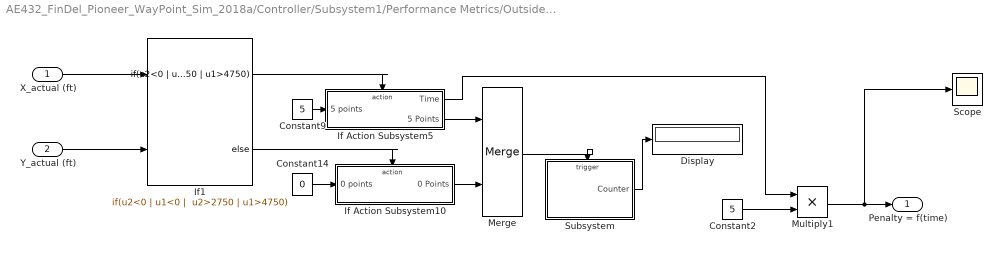
== system AE432_FinDel_Pioneer_WayPoint_Sim_2018a/Controller/Subsystem1/Performance Metrics/Outside Geo-fence ==
  X_actual (ft) : Inport
  Y_actual (ft) : Inport  Port=2
  Constant14 : Constant  Value=0
  Constant2 : Constant  Value=5
  Constant9 : Constant  Value=5
  Display : Display
  If Action Subsystem10 : Subsystem  TreatAsAtomicUnit=on
  If Action Subsystem5 : Subsystem  TreatAsAtomicUnit=on
  If1 : If  NumInputs=2  IfExpression="u2<0 | u1<0 |  u2>2750 | u1>4750"
  Merge : Merge
  Multiply1 : Product
  Scope : Scope
  Subsystem : Subsystem
  Penalty = f(time) : Outport
  wires:
  If1/1 -> If Action Subsystem5/Action
  If1/2 -> If Action Subsystem10/Action
  Constant14/1 -> If Action Subsystem10/1("0 points  ")
  Constant9/1 -> If Action Subsystem5/1("5 points  ")
  If Action Subsystem10/1(0 Points) -> Merge/2
  If Action Subsystem5/2(5 Points) -> Merge/1
  Merge/1 -> Subsystem/Trigger
  Subsystem/1(Counter) -> Display/1
  Constant2/1 -> Multiply1/2
  If Action Subsystem5/1(Time) -> Multiply1/1
  Multiply1/1 -> Scope/1, Penalty = f(time)/1
  X_actual (ft)/1 -> If1/1
  Y_actual (ft)/1 -> If1/2

== system AE432_FinDel_Pioneer_WayPoint_Sim_2018a/Controller/Subsystem1/Performance Metrics/Performance Index Altitude ==
  Z_cmd (ft) : Inport
  Z_actual (ft) : Inport  Port=2
  Add2 : Sum  Inputs=+-
  Constant : Constant  Value=600
  Discrete-Time Integrator2 : DiscreteIntegrator  SampleTime=-1  ICPrevOutput=DiscIntNeverNeededParam  ICPrevScaledInput=DiscIntNeverNeededParam
  Divide2 : Product  Inputs=*/
  Product2 : Product  RndMeth=Zero
  Scope : Scope
  Sqrt2 : Sqrt  SaturateOnIntegerOverflow=on
  Altitude Error : Outport
  wires:
  Product2/1 -> Discrete-Time Integrator2/1
  Divide2/1 -> Sqrt2/1
  Discrete-Time Integrator2/1 -> Divide2/1
  Sqrt2/1 -> Scope/1, Altitude Error/1  "Z"
  Z_cmd (ft)/1 -> Add2/1
  Z_actual (ft)/1 -> Add2/2
  Add2/1 -> Product2/2, Product2/1
  Constant/1 -> Divide2/2
